simulink subsystem "IMUsimulator"  (R2021a)
settings: Solver=VariableStepAuto  StartTime=0.0  StopTime=10.0  RelTol=1e-3
libraries: attitude_library x2
settings Model: Creator=Laura  LastModifiedBy=Laura

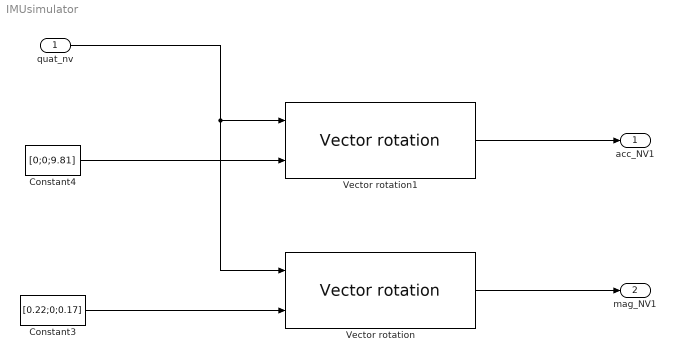
== system IMUsimulator ==
  quat_nv : Inport
  Constant3 : Constant  Value=[0.22;0;0.17]
  Constant4 : Constant  Value=[0;0;9.81]
  Vector rotation : attitude_library/Vector rotation  SystemSampleTime=-1  VariantActivationTime=update diagram  Latency=0  AutoFrameSizeCalculation=off
      settings: SourceProductName=Attitude library
  Vector rotation1 : attitude_library/Vector rotation  SystemSampleTime=-1  VariantActivationTime=update diagram  Latency=0  AutoFrameSizeCalculation=off
      settings: SourceProductName=Attitude library
  acc_NV1 : Outport
  mag_NV1 : Outport  Port=2
  wires:
  quat_nv/1 -> Vector rotation/1, Vector rotation1/1
  Vector rotation/1 -> mag_NV1/1
  Constant3/1 -> Vector rotation/2
  Vector rotation1/1 -> acc_NV1/1
  Constant4/1 -> Vector rotation1/2
